simulink model "Ex4_SoCEstimation"  (R2024b)
settings: Solver=VariableStepAuto  StartTime=0.0  StopTime=3600  RelTol=1e-3
undefined symbols (not defined in the file): Ion, Lithium
libraries: spsBatteryLib x26, spsSeriesRLCBranchLib x3, spsCurrentMeasurementLib x1, spsGroundLib x1, spsSeriesRLCLoadLib x1, spsVoltageMeasurementLib x1, spspowerguiLib x1
settings Model: Creator=balaj  LastModifiedBy=balaj

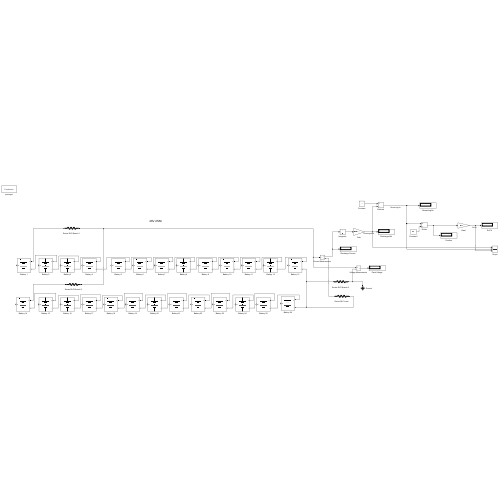
[thumbnail: Simulink's stored preview of the top-level diagram]
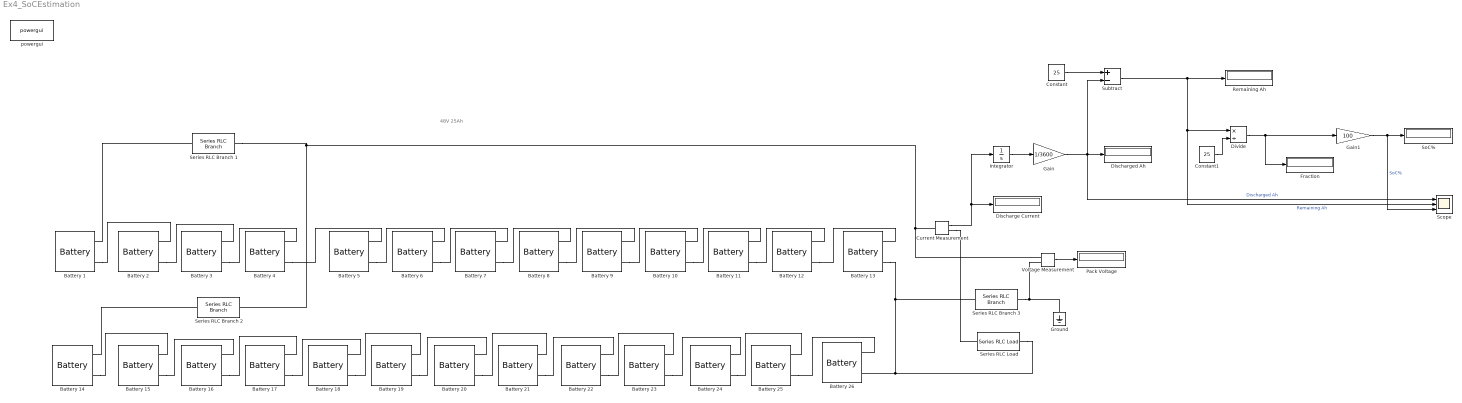
== system Ex4_SoCEstimation ==
  note: 48V 25Ah
  Battery {1..26} (26 alike) : spsBatteryLib/Battery  BatType=Lithium-Ion  NomV=3.7  NomQ=12.5  SOC=100  Batt_Tr=30  PresetModel=on  MaxQ=12.5  MinV=2.775  FullV=4.3068  Dis_rate=5.4348  R=0.00296  Normal_OP=11.3043  expZone="[3.9974     0.61413]"
  Constant : Constant  Value=25
  Constant1 : Constant  Value=25
  "Current Measurement " : spsCurrentMeasurementLib/Current Measurement  PhasorSimulation=off  OutputType=Complex  PSBequivalent=0
  "Discharge Current " : Display
  Discharged Ah : Display
  Divide : Product  Inputs=*/
  Fraction : Display
  Gain : Gain  Gain=1/3600
  Gain1 : Gain  Gain=100
  Ground : spsGroundLib/Ground  LConnTagsString=a
  "Integrator " : Integrator
  Pack Voltage : Display
  Remaining Ah : Display
  Scope : Scope  NumInputPorts=3
  Series RLC Branch 1 : spsSeriesRLCBranchLib/Series RLC Branch  LConnTagsString=__new0  RConnTagsString=__new0  BranchType=R  Resistance=1  Inductance=1e-3  SetiL0=off  InitialCurrent=0  Capacitance=1e-6  Setx0=off  InitialVoltage=0  Measurements=None
  Series RLC Branch 2 : spsSeriesRLCBranchLib/Series RLC Branch  LConnTagsString=__new0  RConnTagsString=__new0  BranchType=R  Resistance=1  Inductance=1e-3  SetiL0=off  InitialCurrent=0  Capacitance=1e-6  Setx0=off  InitialVoltage=0  Measurements=None
  "Series RLC Branch 3 " : spsSeriesRLCBranchLib/Series RLC Branch  LConnTagsString=__new0  RConnTagsString=__new0  BranchType=R  Resistance=1  Inductance=1e-3  SetiL0=off  InitialCurrent=0  Capacitance=1e-6  Setx0=off  InitialVoltage=0  Measurements=None
  "Series RLC Load " : spsSeriesRLCLoadLib/Series RLC Load  LConnTagsString=a  RConnTagsString=__new0  NominalVoltage=48  NominalFrequency=50  ActivePower=1  InductivePower=0  CapacitivePower=0  Setx0=off  InitialVoltage=0  SetiL0=off  InitialCurrent=0  Measurements=None  LoadType=constant Z
  SoC% : Display
  Subtract : Sum  Inputs=+-
  "Voltage Measurement " : spsVoltageMeasurementLib/Voltage Measurement  PhasorSimulation=off  OutputType=Complex  PSBequivalent=0
  powergui : spspowerguiLib/powergui  Priority=1  SimulationMode=Continuous  SampleTime=50e-6  frequency=60  Iterations=50  frequencyindice=0  Pbase=100e6  ErrMax=1e-4  UnitsV=kV  UnitsW=MW  buscounter=0  FunctionMessages=off  echomessages=off  EnableUseOfTLC=off  CurrentSourceSwitches=off  DisableSnubberDevices=off  DisableRonSwitches=off  DisableVfSwitches=off  DisplayEquations=off  AutomaticDiscreteSolvers=off  SolverType=Tustin/Backward Euler (TBE)  Interpol=off  ExternalGateDelay=off  methode=off  Ts=100  x0status=blocks  SPID=on  SwTol=0  HookPort=off  NonlinearTolerance=1e-4  nMaxIteration=100  ContinueOnMaxIteration=off  RestoreLinks=warning  ResistiveCurrentMeasurement=off  Frange=[0:2:500]  Ylog=off  Xlog=on  ShowGrid=off  save=off  variable=ZData  structure=0  ZoomFFT=off  StartTime=0.0  cycles=1  DisplayStyle=1  fundamental=60  FreqAxis=off  MaxFrequency=1000  frequencyindicesteady=1  RmsSteady=1  display=off
  wires:
  "Voltage Measurement "/1 -> Pack Voltage/1
  "Current Measurement "/1 -> "Integrator "/1, "Discharge Current "/1
  Gain1/1 -> Scope/3, SoC%/1  "SoC%"
  Constant/1 -> Subtract/1
  Subtract/1 -> Scope/2, Divide/1, Remaining Ah/1  "Remaining Ah"
  Divide/1 -> Fraction/1, Gain1/1
  Gain/1 -> Scope/1, Subtract/2, Discharged Ah/1  "Discharged Ah"
  Constant1/1 -> Divide/2
  "Integrator "/1 -> Gain/1
  connections:
  Battery 1/LConn2 -- Battery 2/LConn1
  Battery 2/LConn2 -- Battery 3/LConn1
  Battery 3/LConn2 -- Battery 4/LConn1
  Battery 4/LConn2 -- Battery 5/LConn1
  Battery 5/LConn2 -- Battery 6/LConn1
  Battery 6/LConn2 -- Battery 7/LConn1
  Battery 7/LConn2 -- Battery 8/LConn1
  Battery 8/LConn2 -- Battery 9/LConn1
  Battery 9/LConn2 -- Battery 10/LConn1
  Battery 10/LConn2 -- Battery 11/LConn1
  Battery 11/LConn2 -- Battery 12/LConn1
  Battery 12/LConn2 -- Battery 13/LConn1
  Battery 14/LConn2 -- Battery 15/LConn1
  Battery 15/LConn2 -- Battery 16/LConn1
  Battery 16/LConn2 -- Battery 17/LConn1
  Battery 17/LConn2 -- Battery 18/LConn1
  Battery 18/LConn2 -- Battery 19/LConn1
  Battery 19/LConn2 -- Battery 20/LConn1
  Battery 20/LConn2 -- Battery 21/LConn1
  Battery 21/LConn2 -- Battery 22/LConn1
  Battery 22/LConn2 -- Battery 23/LConn1
  Battery 23/LConn2 -- Battery 24/LConn1
  Battery 24/LConn2 -- Battery 25/LConn1
  Battery 25/LConn2 -- Battery 26/LConn1
  Battery 1/LConn1 -- Series RLC Branch 1/LConn1
  Series RLC Branch 2/LConn1 -- Battery 14/LConn1
  Series RLC Branch 1/RConn1 -- "Voltage Measurement "/LConn1 -- "Current Measurement "/LConn1 -- Series RLC Branch 2/RConn1
  "Current Measurement "/RConn1 -- "Series RLC Load "/LConn1
  Battery 13/LConn2 -- Battery 26/LConn2 -- "Series RLC Load "/RConn1 -- "Series RLC Branch 3 "/LConn1
  "Series RLC Branch 3 "/RConn1 -- Ground/LConn1 -- "Voltage Measurement "/LConn2
